simulink model "L05"  (R2021a)
settings: Solver=FixedStepDiscrete  StartTime=0.0  StopTime=60  FixedStep=0.1  RelTol=1e-3
settings Model: EnablePacing=on  PacingRate=3  Creator=ncleju  LastModifiedBy=ncleju
settings OptimizationCC: DefaultParameterBehavior=Inlined  EnhancedBackFolding=on  PassReuseOutputArgsAs=Individual arguments  ZeroExternalMemoryAtStartup=off  ZeroInternalMemoryAtStartup=off  OptimizeBlockOrder=speed  DifferentSizesBufferReuse=on  OptimizationCustomize=off  EfficientTunableParamExpr=on
settings DebuggingCC: ParameterTunabilityLossMsg=error
settings SFSimCC: MATLABDynamicMemAlloc=off
settings RTWCC: SystemTargetFile=ert.tlc  TemplateMakefile=ert_default_tmf
settings CodeAppCC: ForceParamTrailComments=on  IgnoreCustomStorageClasses=off  OperatorAnnotations=on  SimulinkDataObjDesc=on  SFDataObjDesc=on  InsertBlockDesc=on
settings ERTTargetCC: TargetLangStandard=C99 (ISO)  GenerateSampleERTMain=on  InlinedParameterPlacement=NonHierarchical  ERTCustomFileTemplate=example_file_process.tlc

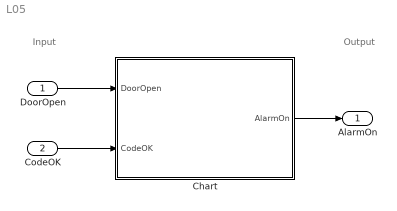
== system L05 ==
  note: Output
  note: Input
  DoorOpen : Inport  OutDataTypeStr=double
  CodeOK : Inport  Port=2
  Chart : Stateflow chart  TreatAsAtomicUnit=on
      settings: RTWSystemCode=Reusable function
  AlarmOn : Outport
  wires:
  DoorOpen/1 -> Chart/1(DoorOpen)
  CodeOK/1 -> Chart/2(CodeOK)
  Chart/1(AlarmOn) -> AlarmOn/1

== stateflow chart L05/Chart ==
  state ALARM_ARMED
    en:
    AlarmOn = false;
  state ALARM_DISARMED
    en:
    AlarmOn = false;
  state DOOR_OPEN
    state WAIT_15_SEC
    state ALARM_ON
      en:
      AlarmOn = true;
    WAIT_15_SEC -> ALARM_ON : [after(150, tick)]
  (default) -> ALARM_ARMED
  ALARM_DISARMED -> ALARM_ARMED : [DoorOpen == false]
  ALARM_ARMED -> WAIT_15_SEC : [DoorOpen == true]
  DOOR_OPEN -> ALARM_DISARMED : [CodeOK == true]
  data: DoorOpen input; CodeOK input; AlarmOn output
